simulink model "lab3CTSys2"  (R2021b)
settings: Solver=ode45  StartTime=0.0  StopTime=10  MaxStep=.05  RelTol=1e-3  AbsTol=1e-6
settings Model: Creator=vise  LastModifiedBy=ishau
settings SolverCC: AutoScaleAbsTol=off  AlgebraicLoopSolver=TrustRegion
settings DataIOCC: SaveFormat=Array  SignalLoggingSaveFormat=ModelDataLogs  ReturnWorkspaceOutputs=off
settings OptimizationCC: BooleanDataType=off  ExpressionDepthLimit=2147483647  InitFltsAndDblsToZero=on  LifeSpan=inf
settings DebuggingCC: SaveWithParameterizedLinksMsg=none  UnderspecifiedInitializationDetection=Classic  MergeDetectMultiDrivingBlocksExec=none  SignalResolutionControl=TryResolveAllWithWarning  MultiTaskDSMMsg=warning  MultiTaskCondExecSysMsg=none  FcnCallInpInsideContextMsg=warning  StateNameClashWarn=warning  SFUnexpectedBacktrackingDiag=warning  SFNoUnconditionalDefaultTransitionDiag=warning  SFExecutionAtInitializationDiag=none  SFMachineParentedDataDiag=warning  ArithmeticOperatorsInVariantConditions=warning
settings HardwareCC: ProdBitPerPointer=32  ProdBitPerSizeT=32  ProdBitPerPtrDiffT=32  ProdLargestAtomicFloat=None  ProdIntDivRoundTo=Undefined  ProdEndianess=Unspecified  ProdWordSize=32  ProdHWDeviceType=32-bit Generic  TargetUnknown=on
settings ModelReferenceCC: PropagateSignalLabelsOutOfModel=off
settings SFSimCC: SimUseLocalCustomCode=off  CustomCodeUndefinedFunction=UseInterfaceOnly
settings RTWCC: TemplateMakefile=grt_unix.tmf  RTWUseLocalCustomCode=off
settings CodeAppCC: StateflowObjectComments=on
settings GRTTargetCC: TargetLangStandard=C89/C90 (ANSI)  CombineOutputUpdateFcns=off  GRTInterface=on
settings ConfigComp: CovMetricSettings=dw  CovSaveCumulativeToWorkspaceVar=on  CovSaveSingleToWorkspaceVar=on  CovExternalEMLEnable=off

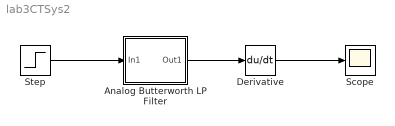
== system lab3CTSys2 ==
  Analog Butterworth LP Filter : Subsystem  mask(buttap){MaskParam1=2*pi, MaskParam2=4}
      mask prompts: MaskParam1 "Cutoff frequency (rad/sec)"; MaskParam2 "Order"
      mask help:
      | Analog Butterworth low pass filter.
      |
      | (Requires Signal Processing Toolbox)
      mask init:
      | [z,p,k]=buttap(MaskParam2); z=MaskParam1*z; p=MaskParam1*p; k=real(prod(-p)); [num,den]=zp2tf(z,p,k); w=logspace(log10(MaskParam1/10),log10(10*MaskParam1),20); h=freqs(num,den,w);
      mask Help: Butterworth low pass filter using MATLAB's butter command.
      mask Display: plot(20*log10(w),20*log10(abs(h)))
  Derivative : Derivative
  Scope : Scope
  Step : Step  Time=0.00001  SampleTime=0
  wires:
  Analog Butterworth LP Filter/1(Out1) -> Derivative/1
  Step/1 -> Analog Butterworth LP Filter/1(In1)
  Derivative/1 -> Scope/1

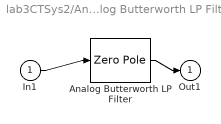
== system lab3CTSys2/Analog Butterworth LP Filter ==
  In1 : Inport
  Analog Butterworth LP Filter : ZeroPole  Zeros=z  Poles=p  Gain=k
  Out1 : Outport
  wires:
  In1/1 -> Analog Butterworth LP Filter/1
  Analog Butterworth LP Filter/1 -> Out1/1
